simulink model "Ejercicio_Propuesto_1"  (R2023a)
settings: Solver=VariableStepAuto  StartTime=0.0  StopTime=10.0  RelTol=1e-3
values from neighbouring files (symbols this model uses):
  a = 1/(A*B)    (= 50000)    [Ejercicio_1.m]
  b = 1/B    (= 10000)    [Ejercicio_1.m]
  K = 100    [Ejercicio_1.m]    (also in Ejercicio_Propuesto_1_y_3.m = 1)
  s = 1    [Ejercicio_1.m]
settings Model: Creator=laura  LastModifiedBy=laura

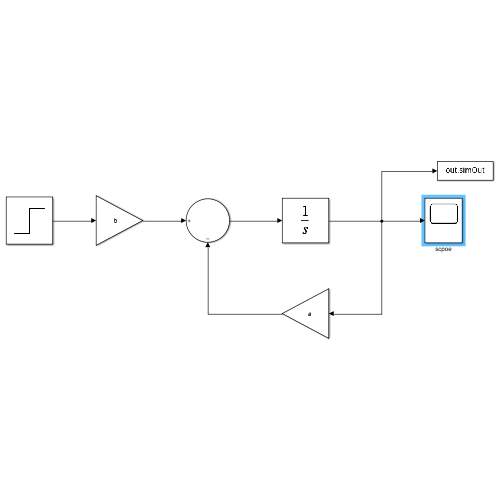
[thumbnail: Simulink's stored preview of the top-level diagram]
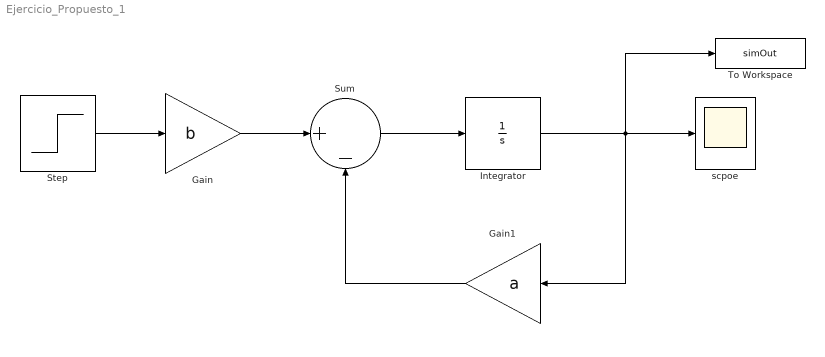
== system Ejercicio_Propuesto_1 ==
  Gain : Gain  Gain=b
  Gain1 : Gain  Gain=a
  Integrator : Integrator
  Step : Step  Time=s  After=K  SampleTime=0
  Sum : Sum  Inputs=|+-
  To Workspace : ToWorkspace  VariableName=simOut  SaveFormat=Timeseries  SampleTime=-1
  scpoe : Scope
  wires:
  Integrator/1 -> To Workspace/1, scpoe/1, Gain1/1
  Step/1 -> Gain/1
  Gain/1 -> Sum/1
  Sum/1 -> Integrator/1
  Gain1/1 -> Sum/2
